simulink model "engineMassModel"  (R2020a)
settings: Solver=VariableStepAuto  StartTime=0.0  StopTime=10.0  RelTol=1e-3
values from neighbouring files (symbols this model uses):
  average_rho = (LOX_rho*LOX_l + fuel_rho*fuel_l)/(LOX_l+fuel_l)    (= 1.01371428571)    [engineMassModelM.m]
  flowrate_gain = 0.000042386326    (= 4.2386326e-05)    [engineMassModelM.m]
  flowrate_offset = 0.02812874067    [engineMassModelM.m]
  m_i = LOX_m_i + fuel_m_i    [engineMassModelM.m]
  mil_to_cu_in = 0.0610237    [engineMassModelM.m]
  p_i = 1000    [engineMassModelM.m]
  press_vol = press_l * pi() * (tube_id/2)^2    [engineMassModelM.m]
undefined symbols (not defined in the file or in its folder): prop_mass_i
settings Model: Creator=Makar  LastModifiedBy=Makar

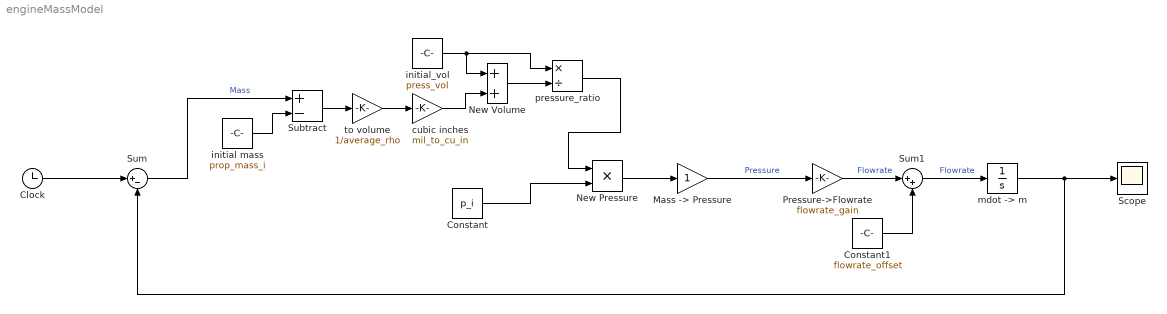
== system engineMassModel ==
  Clock : Clock
  Constant : Constant  Value=p_i
  Constant1 : Constant  Value=flowrate_offset
  "Mass -> Pressure" : Gain
  New Pressure : Product  Inputs=**
  New Volume : Sum
  Pressure->Flowrate : Gain  Gain=flowrate_gain
  Scope : Scope
  Subtract : Sum  Inputs=+-
  Sum : Sum  Inputs=|+-
  Sum1 : Sum  Inputs=|++
  cubic inches : Gain  Gain=mil_to_cu_in
  initial mass : Constant  Value=prop_mass_i
  initial_vol : Constant  Value=press_vol
  "mdot -> m" : Integrator  InitialCondition=m_i
  pressure_ratio : Product  Inputs=*/
  to volume : Gain  Gain=1/average_rho
  wires:
  Sum/1 -> Subtract/1  "Mass"
  "Mass -> Pressure"/1 -> Pressure->Flowrate/1  "Pressure"
  Sum1/1 -> "mdot -> m"/1  "Flowrate"
  "mdot -> m"/1 -> Scope/1, Sum/2
  initial mass/1 -> Subtract/2
  Subtract/1 -> to volume/1
  to volume/1 -> cubic inches/1
  cubic inches/1 -> New Volume/2
  initial_vol/1 -> pressure_ratio/1, New Volume/1
  New Volume/1 -> pressure_ratio/2
  New Pressure/1 -> "Mass -> Pressure"/1
  pressure_ratio/1 -> New Pressure/1
  Constant/1 -> New Pressure/2
  Pressure->Flowrate/1 -> Sum1/1  "Flowrate"
  Constant1/1 -> Sum1/2
  Clock/1 -> Sum/1
